simulink model "plantsimulation"  (R2018a)
settings: Solver=VariableStepAuto  StartTime=0.0  StopTime=10.0  RelTol=1e-3
libraries: cstblocks x3
settings Model: Creator=nigam4  LastModifiedBy=nigam4

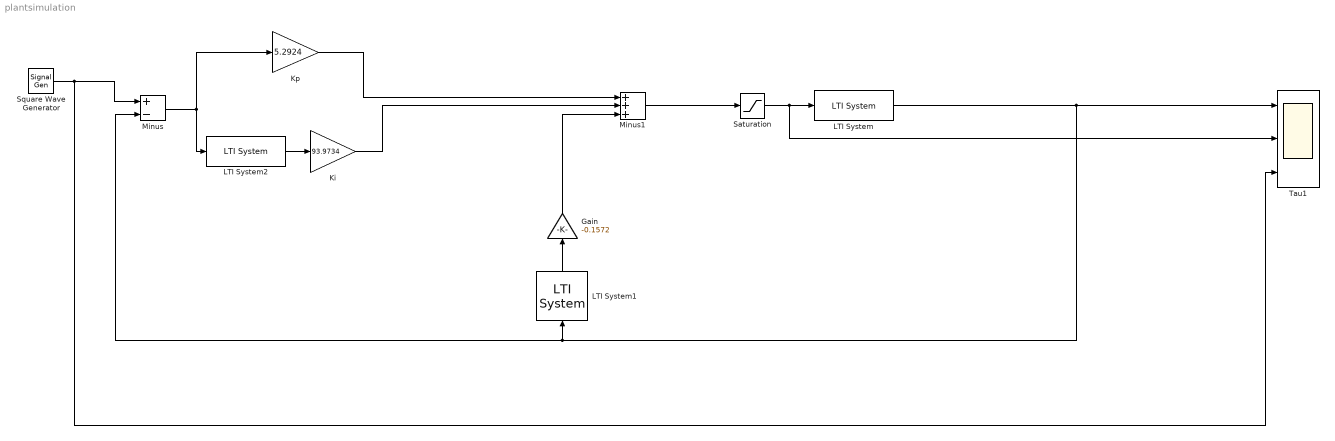
== system plantsimulation ==
  Gain : Gain  Gain=-0.1572
  Ki : Gain  Gain=93.9734
  Kp : Gain  Gain=5.2924
  LTI System : cstblocks/LTI System  sys=plantdtf  IC=[]
  LTI System1 : cstblocks/LTI System  sys=Ddtf  IC=[]
  LTI System2 : cstblocks/LTI System  sys=ditf  IC=[]
  Minus : Sum  Inputs=+-
  Minus1 : Sum  Inputs=+++
  Saturation : Saturate  UpperLimit=10  LowerLimit=-10
  Square Wave Generator : SignalGenerator  WaveForm=square  Amplitude=-3  Frequency=1/30
  Tau1 : Scope  NumInputPorts=3
  wires:
  Minus1/1 -> Saturation/1
  Kp/1 -> Minus1/1
  Ki/1 -> Minus1/2
  Saturation/1 -> Tau1/2, LTI System/1
  Minus/1 -> LTI System2/1, Kp/1
  LTI System/1 -> Minus/2, LTI System1/1, Tau1/1
  LTI System1/1 -> Gain/1
  Gain/1 -> Minus1/3
  LTI System2/1 -> Ki/1
  Square Wave Generator/1 -> Tau1/3, Minus/1
